simulink model "z_compare"  (R2018a)
settings: Solver=VariableStepAuto  StartTime=0.0  StopTime=20  RelTol=1e-3
undefined symbols (not defined in the file): drone, est_c_A, est_c_B, est_c_C, est_c_D, simulation_sampling_ts
libraries: simulink x5
settings Model: Creator=ros  LastModifiedBy=ros

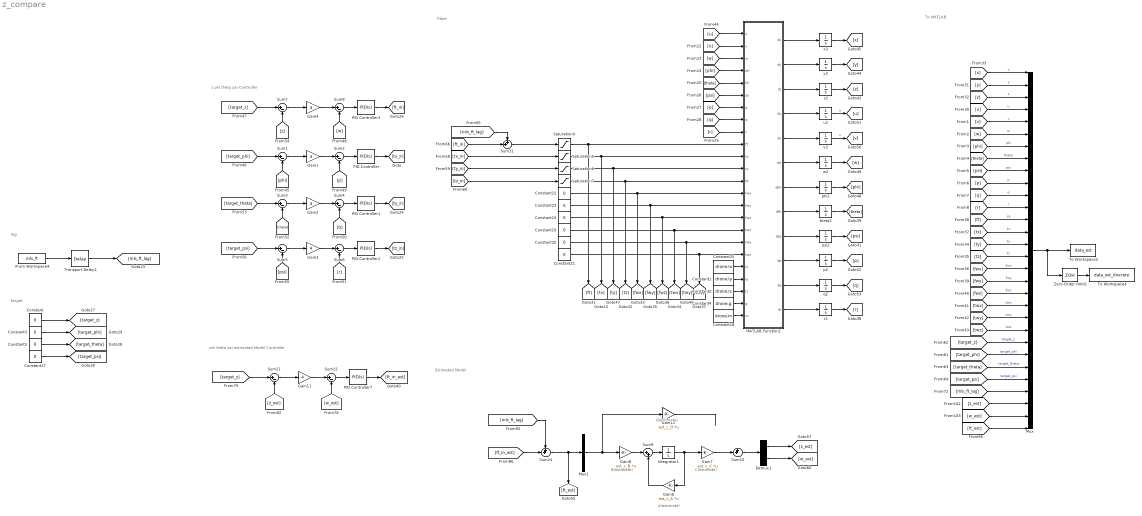
== system z_compare ==
  note: B(estimate)
  note: C(estimate)
  note: A(estimate)
  note: D(estimate)
  note: Plant
  note: To MATLAB
  note: Estimated Model
  note: lag
  note: target
  note: z phi theta psi Controller
  note: phi theta psi estimated Model Controller
  Constant{,3,5,17,19..24} (10 alike) : Constant  Value=0
  Constant1 : Constant  Value=drone.Iy
  Constant18 : Constant  Value=drone.m
  Constant2 : Constant  Value=drone.Iz
  Constant25 : Constant  Value=drone.Ix
  Constant4 : Constant  Value=drone.g
  Demux1 : Demux  Outputs=2
  From Workspace4 : FromWorkspace  VariableName=mls_ft  SampleTime=0
  Gain{1..4,11} (5 alike) : Gain  Gain=4
  Gain12 : Gain  Gain=est_c_D  Multiplication=Matrix(K*u)
  Gain6 : Gain  Gain=est_c_A  Multiplication=Matrix(K*u)
  Gain7 : Gain  Gain=est_c_C  Multiplication=Matrix(K*u)
  Gain8 : Gain  Gain=est_c_B  Multiplication=Matrix(K*u)
  Integrator1 : Integrator
  MATLAB Function1 : MATLAB Function  TreatAsAtomicUnit=on
  Mux : Mux  Inputs=30
  Mux1 : Mux  Inputs=1
  PID Controller : simulink/Continuous/PID Controller  Controller=PID  TimeDomain=Continuous-time  SampleTime=-1  IntegratorMethod=Forward Euler  FilterMethod=Forward Euler  Form=Parallel  UseFilter=on  ControllerParametersSource=internal  P=1.5  I=1.5  D=0  N=100  InitialConditionSource=internal  InitialConditionForIntegrator=0  InitialConditionForFilter=0  ExternalReset=none  LimitOutput=off  UpperSaturationLimit=inf  LowerSaturationLimit=-inf  LinearizeAsGain=on  AntiWindupMode=none  Kb=1  TrackingMode=off  Kt=1  PParamMin=[]  PParamMax=[]  IParamMin=[]  IParamMax=[]  DParamMin=[]  DParamMax=[]  NParamMin=[]  NParamMax=[]  KbParamMin=[]  KbParamMax=[]  KtParamMin=[]  KtParamMax=[]  POutMin=[]  POutMax=[]  IOutMin=[]  IOutMax=[]  DOutMin=[]  DOutMax=[]  NOutMin=[]  NOutMax=[]  KbOutMin=[]  KbOutMax=[]  KtOutMin=[]  KtOutMax=[]  IntegratorOutMin=[]  IntegratorOutMax=[]  FilterOutMin=[]  FilterOutMax=[]  SumOutMin=[]  SumOutMax=[]  SumI1OutMin=[]  SumI1OutMax=[]  SumI2OutMin=[]  SumI2OutMax=[]  SumI3OutMin=[]  SumI3OutMax=[]  SumDOutMin=[]  SumDOutMax=[]  SaturationOutMin=[]  SaturationOutMax=[]  IntegratorContinuousStateAttributes=''  IntegratorStateMustResolveToSignalObject=off  IntegratorRTWStateStorageClass=Auto  FilterContinuousStateAttributes=''  FilterStateMustResolveToSignalObject=off  FilterRTWStateStorageClass=Auto  DifferentiatorICPrevScaledInput=0  DifferentiatorOutMin=[]  DifferentiatorOutMax=[]  FilterDiffOutCoefMin=[]  FilterDiffOutCoefMax=[]  SumDenOutMin=[]  SumDenOutMax=[]  SumNumOutMin=[]  SumNumOutMax=[]  ReciprocalOutMin=[]  ReciprocalOutMax=[]  DivideOutMin=[]  DivideOutMax=[]  TunerSelectOption=Transfer Function Based (PID Tuner App)
  PID Controller1 : simulink/Continuous/PID Controller  Controller=PID  TimeDomain=Continuous-time  SampleTime=-1  IntegratorMethod=Forward Euler  FilterMethod=Forward Euler  Form=Parallel  UseFilter=on  ControllerParametersSource=internal  P=1.5  I=1.5  D=0  N=100  InitialConditionSource=internal  InitialConditionForIntegrator=0  InitialConditionForFilter=0  ExternalReset=none  LimitOutput=off  UpperSaturationLimit=inf  LowerSaturationLimit=-inf  LinearizeAsGain=on  AntiWindupMode=none  Kb=1  TrackingMode=off  Kt=1  PParamMin=[]  PParamMax=[]  IParamMin=[]  IParamMax=[]  DParamMin=[]  DParamMax=[]  NParamMin=[]  NParamMax=[]  KbParamMin=[]  KbParamMax=[]  KtParamMin=[]  KtParamMax=[]  POutMin=[]  POutMax=[]  IOutMin=[]  IOutMax=[]  DOutMin=[]  DOutMax=[]  NOutMin=[]  NOutMax=[]  KbOutMin=[]  KbOutMax=[]  KtOutMin=[]  KtOutMax=[]  IntegratorOutMin=[]  IntegratorOutMax=[]  FilterOutMin=[]  FilterOutMax=[]  SumOutMin=[]  SumOutMax=[]  SumI1OutMin=[]  SumI1OutMax=[]  SumI2OutMin=[]  SumI2OutMax=[]  SumI3OutMin=[]  SumI3OutMax=[]  SumDOutMin=[]  SumDOutMax=[]  SaturationOutMin=[]  SaturationOutMax=[]  IntegratorContinuousStateAttributes=''  IntegratorStateMustResolveToSignalObject=off  IntegratorRTWStateStorageClass=Auto  FilterContinuousStateAttributes=''  FilterStateMustResolveToSignalObject=off  FilterRTWStateStorageClass=Auto  DifferentiatorICPrevScaledInput=0  DifferentiatorOutMin=[]  DifferentiatorOutMax=[]  FilterDiffOutCoefMin=[]  FilterDiffOutCoefMax=[]  SumDenOutMin=[]  SumDenOutMax=[]  SumNumOutMin=[]  SumNumOutMax=[]  ReciprocalOutMin=[]  ReciprocalOutMax=[]  DivideOutMin=[]  DivideOutMax=[]  TunerSelectOption=Transfer Function Based (PID Tuner App)
  PID Controller2 : simulink/Continuous/PID Controller  Controller=PID  TimeDomain=Continuous-time  SampleTime=-1  IntegratorMethod=Forward Euler  FilterMethod=Forward Euler  Form=Parallel  UseFilter=on  ControllerParametersSource=internal  P=1.5  I=1.5  D=0  N=100  InitialConditionSource=internal  InitialConditionForIntegrator=0  InitialConditionForFilter=0  ExternalReset=none  LimitOutput=off  UpperSaturationLimit=inf  LowerSaturationLimit=-inf  LinearizeAsGain=on  AntiWindupMode=none  Kb=1  TrackingMode=off  Kt=1  PParamMin=[]  PParamMax=[]  IParamMin=[]  IParamMax=[]  DParamMin=[]  DParamMax=[]  NParamMin=[]  NParamMax=[]  KbParamMin=[]  KbParamMax=[]  KtParamMin=[]  KtParamMax=[]  POutMin=[]  POutMax=[]  IOutMin=[]  IOutMax=[]  DOutMin=[]  DOutMax=[]  NOutMin=[]  NOutMax=[]  KbOutMin=[]  KbOutMax=[]  KtOutMin=[]  KtOutMax=[]  IntegratorOutMin=[]  IntegratorOutMax=[]  FilterOutMin=[]  FilterOutMax=[]  SumOutMin=[]  SumOutMax=[]  SumI1OutMin=[]  SumI1OutMax=[]  SumI2OutMin=[]  SumI2OutMax=[]  SumI3OutMin=[]  SumI3OutMax=[]  SumDOutMin=[]  SumDOutMax=[]  SaturationOutMin=[]  SaturationOutMax=[]  IntegratorContinuousStateAttributes=''  IntegratorStateMustResolveToSignalObject=off  IntegratorRTWStateStorageClass=Auto  FilterContinuousStateAttributes=''  FilterStateMustResolveToSignalObject=off  FilterRTWStateStorageClass=Auto  DifferentiatorICPrevScaledInput=0  DifferentiatorOutMin=[]  DifferentiatorOutMax=[]  FilterDiffOutCoefMin=[]  FilterDiffOutCoefMax=[]  SumDenOutMin=[]  SumDenOutMax=[]  SumNumOutMin=[]  SumNumOutMax=[]  ReciprocalOutMin=[]  ReciprocalOutMax=[]  DivideOutMin=[]  DivideOutMax=[]  TunerSelectOption=Transfer Function Based (PID Tuner App)
  PID Controller3 : simulink/Continuous/PID Controller  Controller=PID  TimeDomain=Continuous-time  SampleTime=-1  IntegratorMethod=Forward Euler  FilterMethod=Forward Euler  Form=Parallel  UseFilter=on  ControllerParametersSource=internal  P=7  I=6  D=0.7  N=100  InitialConditionSource=internal  InitialConditionForIntegrator=0  InitialConditionForFilter=0  ExternalReset=none  LimitOutput=off  UpperSaturationLimit=inf  LowerSaturationLimit=-inf  LinearizeAsGain=on  AntiWindupMode=none  Kb=1  TrackingMode=off  Kt=1  PParamMin=[]  PParamMax=[]  IParamMin=[]  IParamMax=[]  DParamMin=[]  DParamMax=[]  NParamMin=[]  NParamMax=[]  KbParamMin=[]  KbParamMax=[]  KtParamMin=[]  KtParamMax=[]  POutMin=[]  POutMax=[]  IOutMin=[]  IOutMax=[]  DOutMin=[]  DOutMax=[]  NOutMin=[]  NOutMax=[]  KbOutMin=[]  KbOutMax=[]  KtOutMin=[]  KtOutMax=[]  IntegratorOutMin=[]  IntegratorOutMax=[]  FilterOutMin=[]  FilterOutMax=[]  SumOutMin=[]  SumOutMax=[]  SumI1OutMin=[]  SumI1OutMax=[]  SumI2OutMin=[]  SumI2OutMax=[]  SumI3OutMin=[]  SumI3OutMax=[]  SumDOutMin=[]  SumDOutMax=[]  SaturationOutMin=[]  SaturationOutMax=[]  IntegratorContinuousStateAttributes=''  IntegratorStateMustResolveToSignalObject=off  IntegratorRTWStateStorageClass=Auto  FilterContinuousStateAttributes=''  FilterStateMustResolveToSignalObject=off  FilterRTWStateStorageClass=Auto  DifferentiatorICPrevScaledInput=0  DifferentiatorOutMin=[]  DifferentiatorOutMax=[]  FilterDiffOutCoefMin=[]  FilterDiffOutCoefMax=[]  SumDenOutMin=[]  SumDenOutMax=[]  SumNumOutMin=[]  SumNumOutMax=[]  ReciprocalOutMin=[]  ReciprocalOutMax=[]  DivideOutMin=[]  DivideOutMax=[]  TunerSelectOption=Transfer Function Based (PID Tuner App)
  PID Controller7 : simulink/Continuous/PID Controller  Controller=PID  TimeDomain=Continuous-time  SampleTime=-1  IntegratorMethod=Forward Euler  FilterMethod=Forward Euler  Form=Parallel  UseFilter=on  ControllerParametersSource=internal  P=7  I=6  D=0.7  N=100  InitialConditionSource=internal  InitialConditionForIntegrator=0  InitialConditionForFilter=0  ExternalReset=none  LimitOutput=off  UpperSaturationLimit=inf  LowerSaturationLimit=-inf  LinearizeAsGain=on  AntiWindupMode=none  Kb=1  TrackingMode=off  Kt=1  PParamMin=[]  PParamMax=[]  IParamMin=[]  IParamMax=[]  DParamMin=[]  DParamMax=[]  NParamMin=[]  NParamMax=[]  KbParamMin=[]  KbParamMax=[]  KtParamMin=[]  KtParamMax=[]  POutMin=[]  POutMax=[]  IOutMin=[]  IOutMax=[]  DOutMin=[]  DOutMax=[]  NOutMin=[]  NOutMax=[]  KbOutMin=[]  KbOutMax=[]  KtOutMin=[]  KtOutMax=[]  IntegratorOutMin=[]  IntegratorOutMax=[]  FilterOutMin=[]  FilterOutMax=[]  SumOutMin=[]  SumOutMax=[]  SumI1OutMin=[]  SumI1OutMax=[]  SumI2OutMin=[]  SumI2OutMax=[]  SumI3OutMin=[]  SumI3OutMax=[]  SumDOutMin=[]  SumDOutMax=[]  SaturationOutMin=[]  SaturationOutMax=[]  IntegratorContinuousStateAttributes=''  IntegratorStateMustResolveToSignalObject=off  IntegratorRTWStateStorageClass=Auto  FilterContinuousStateAttributes=''  FilterStateMustResolveToSignalObject=off  FilterRTWStateStorageClass=Auto  DifferentiatorICPrevScaledInput=0  DifferentiatorOutMin=[]  DifferentiatorOutMax=[]  FilterDiffOutCoefMin=[]  FilterDiffOutCoefMax=[]  SumDenOutMin=[]  SumDenOutMax=[]  SumNumOutMin=[]  SumNumOutMax=[]  ReciprocalOutMin=[]  ReciprocalOutMax=[]  DivideOutMin=[]  DivideOutMax=[]  TunerSelectOption=Transfer Function Based (PID Tuner App)
  Saturation{4..7} (4 alike) : Saturate  UpperLimit=30  LowerLimit=-100
  Sum{1..8,21..22} (10 alike) : Sum  Inputs=|+-
  Sum10 : Sum  Inputs=++|
  Sum11 : Sum  Inputs=++|
  Sum24 : Sum  Inputs=++|
  Sum9 : Sum  Inputs=|++
  To Workspace2 : ToWorkspace  VariableName=data_est  SaveFormat=Timeseries  SampleTime=-1
  To Workspace4 : ToWorkspace  VariableName=data_est_discrete  SaveFormat=Timeseries  SampleTime=-1
  Transport Delay4 : TransportDelay  DelayTime=10
  Zero-Order Hold1 : ZeroOrderHold  SampleTime=simulation_sampling_ts
  p2 : Integrator
  phi2 : Integrator
  psi2 : Integrator
  q2 : Integrator
  r2 : Integrator
  theta2 : Integrator
  u2 : Integrator
  v2 : Integrator
  w2 : Integrator
  x2 : Integrator
  y2 : Integrator
  z2 : Integrator
  wires:
  [x] -> Mux/1  "x"
  [v] -> Mux/5  "v"
  [z] -> Mux/3  "z"
  [w] -> Mux/6  "w"
  [p] -> Mux/10  "p"
  [phi] -> Mux/7  "phi"
  [theta] -> Mux/8  "theta"
  [r] -> Mux/12  "r"
  [y] -> Mux/2  "y"
  [psi] -> Mux/9  "psi"
  [u] -> Mux/4  "u"
  [q] -> Mux/11  "q"
  Mux/1 -> Zero-Order Hold1/1, To Workspace2/1
  [ft] -> Mux/13  "ft"
  [tx] -> Mux/14  "tx"
  [ty] -> Mux/15  "ty"
  [tz] -> Mux/16  "tz"
  [fwx] -> Mux/17  "fwx"
  [fwy] -> Mux/18  "fwy"
  [fwz] -> Mux/19  "fwz"
  [twx] -> Mux/20  "twx"
  [twy] -> Mux/21  "twy"
  [twz] -> Mux/22  "twz"
  Zero-Order Hold1/1 -> To Workspace4/1
  [phi] -> Sum1/2
  [target_phi] -> Sum1/1
  Sum1/1 -> Gain1/1
  Gain1/1 -> Sum2/1
  Sum2/1 -> PID Controller/1
  [p] -> Sum2/2
  [q] -> Sum4/2
  Gain2/1 -> Sum4/1
  [target_theta] -> Sum3/1
  Sum4/1 -> PID Controller1/1
  Sum3/1 -> Gain2/1
  [theta] -> Sum3/2
  [r] -> Sum6/2
  Gain3/1 -> Sum6/1
  [target_psi] -> Sum5/1
  Sum6/1 -> PID Controller2/1
  Sum5/1 -> Gain3/1
  [psi] -> Sum5/2
  [target_z] -> Sum7/1
  Sum8/1 -> PID Controller3/1
  [w] -> Sum8/2
  Sum7/1 -> Gain4/1
  Gain4/1 -> Sum8/1
  [z] -> Sum7/2
  PID Controller/1 -> [tx_in]
  PID Controller2/1 -> [tz_in]
  PID Controller1/1 -> [ty_in]
  PID Controller3/1 -> [ft_in]
  [target_z] -> Mux/23  "target_z"
  [target_phi] -> Mux/24  "target_phi"
  [target_theta] -> Mux/25  "target_theta"
  [target_psi] -> Mux/26  "target_psi"
  Constant17/1 -> [target_psi]
  Constant5/1 -> [target_theta]
  Constant/1 -> [target_z]
  Constant3/1 -> [target_phi]
  Mux1/1 -> Gain12/1, Gain8/1
  Sum9/1 -> Integrator1/1
  Integrator1/1 -> Gain7/1, Gain6/1
  Gain8/1 -> Sum9/1
  Gain6/1 -> Sum9/2
  Gain7/1 -> Sum10/2
  Gain12/1 -> ?
  Sum10/1 -> Demux1/1
  [mls_ft_lag] -> Sum24/1
  Sum24/1 -> [ft_est], Mux1/1
  [ft_in_est] -> Sum24/2
  [mls_ft_lag] -> Mux/27
  From Workspace4/1 -> Transport Delay4/1
  Transport Delay4/1 -> [mls_ft_lag]
  Sum22/1 -> PID Controller7/1
  Gain11/1 -> Sum22/1
  Sum21/1 -> Gain11/1
  PID Controller7/1 -> [ft_in_est]
  [z_est] -> Sum21/2
  [target_z] -> Sum21/1
  [w_est] -> Sum22/2
  Demux1/1 -> [z_est]
  Demux1/2 -> [w_est]
  [z_est] -> Mux/28
  [w_est] -> Mux/29
  [ft_est] -> Mux/30
  [v] -> MATLAB Function1/2(v)
  [r] -> MATLAB Function1/9(r)
  Constant18/1 -> MATLAB Function1/24(m)
  Constant23/1 -> [fwy], MATLAB Function1/15(fwy)
  MATLAB Function1/7(dph) -> phi2/1
  [psi] -> MATLAB Function1/6(ps)
  MATLAB Function1/12(dr) -> r2/1
  Saturation5/1 -> [tx], MATLAB Function1/11(tx)
  [w] -> MATLAB Function1/3(w)
  theta2/1 -> [theta]
  MATLAB Function1/6(dw) -> w2/1
  [q] -> MATLAB Function1/8(q)
  Sum11/1 -> Saturation4/1
  [phi] -> MATLAB Function1/4(ph)
  u2/1 -> [u]  "u"
  z2/1 -> [z]
  [ty_in] -> Saturation6/1
  MATLAB Function1/5(dv) -> v2/1
  q2/1 -> [q]
  [ft_in] -> Sum11/2
  [tx_in] -> Saturation5/1
  Saturation6/1 -> [ty], MATLAB Function1/12(ty)
  x2/1 -> [x]
  p2/1 -> [p]
  Constant19/1 -> [twx], MATLAB Function1/17(twx)
  MATLAB Function1/3(dz) -> z2/1
  [u] -> MATLAB Function1/1(u)
  [tz_in] -> Saturation7/1
  MATLAB Function1/10(dp) -> p2/1
  v2/1 -> [v]  "v"
  [mls_ft_lag] -> Sum11/1
  MATLAB Function1/4(du) -> u2/1
  MATLAB Function1/11(dq) -> q2/1
  Saturation7/1 -> [tz], MATLAB Function1/13(tz)
  Constant21/1 -> [twz], MATLAB Function1/19(twz)
  Constant1/1 -> MATLAB Function1/21(Iy)
  w2/1 -> [w]
  MATLAB Function1/2(dy) -> y2/1
  Saturation4/1 -> [ft], MATLAB Function1/10(ft)
  [theta] -> MATLAB Function1/5(th)
  MATLAB Function1/1(dx) -> x2/1
  r2/1 -> [r]
  Constant4/1 -> MATLAB Function1/23(g)
  Constant22/1 -> [fwx], MATLAB Function1/14(fwx)
  phi2/1 -> [phi]
  Constant2/1 -> MATLAB Function1/22(Iz)
  psi2/1 -> [psi]
  Constant24/1 -> [fwz], MATLAB Function1/16(fwz)
  y2/1 -> [y]
  Constant25/1 -> MATLAB Function1/20(Ix)
  [p] -> MATLAB Function1/7(p)
  MATLAB Function1/9(dps) -> psi2/1
  Constant20/1 -> [twy], MATLAB Function1/18(twy)
  MATLAB Function1/8(dth) -> theta2/1

== matlab function z_compare/MATLAB Function1 ==
  data: u input; v input; dx output; w input; ph input; th input; ps input; p input; q input; r input; ft input; tx input; ty input; tz input; fwx input; fwy input; fwz input; twx input; twy input; twz input; dy output; dz output; du output; dv output; dw output; dph output; dth output; dps output; dp output; dq output; dr output; Ix input; Iy input; Iz input; g input; m input
function [dx, dy, dz, du, dv, dw, dph, dth, dps, dp, dq, dr] = fcn(u, v, w, ph, th, ps, p, q, r, ft, tx, ty, tz, fwx, fwy, fwz, twx, twy, twz, Ix, Iy, Iz, g, m)

dx = w*(sin(ph)*sin(ps) + cos(ph)*cos(ps)*sin(th)) - v*(cos(ph)*sin(ps) - cos(ps)*sin(ph)*sin(th)) + u*(cos(ps)*cos(th));
dy = v*(cos(ph)*cos(ps) + sin(ph)*sin(ps)*sin(th)) - w*(cos(ps)*sin(ph) - cos(ph)*sin(ps)*sin(th)) + u*(cos(th)*sin(ps));
dz = w*(cos(ph)*cos(th)) - u*(sin(th)) + v*(cos(th)*sin(ph));
du = r*v - q*w + g*(sin(th)) + fwx / m;
dv = p*w - r*u - g*(sin(ph)*cos(th)) + fwy / m;
dw = q*u - p*v - g*(cos(th)*cos(ph)) + (fwz + ft) / m;
dph = p + r*(cos(ph)*tan(th)) + q*(sin(ph)*tan(th));
dth = q*(cos(th)) - r*(sin(ph));
dps = r*(cos(ph)/cos(th)) + q*(sin(ph)/cos(th));
dp = r*q*(Iy - Iz)/Ix + (tx + twx)/Ix;
dq = p*r*(Iz - Ix)/Iy + (ty + twy)/Iy;
dr = p*q*(Ix - Iy)/Iz + (tz + twz)/Iz;
